simulink model "TrafficLightSystem_PhyArch_Electrical"  (R2025b)
settings: Solver=VariableStepAuto  StartTime=0.0  StopTime=10.0  RelTol=1e-3
settings Model: Creator=maric  LastModifiedBy=maric

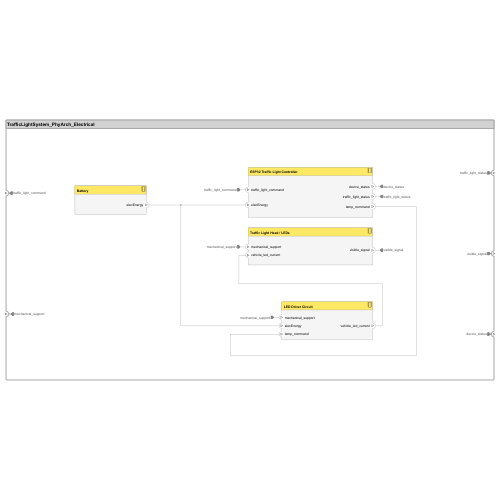
[thumbnail: Simulink's stored preview of the top-level diagram]
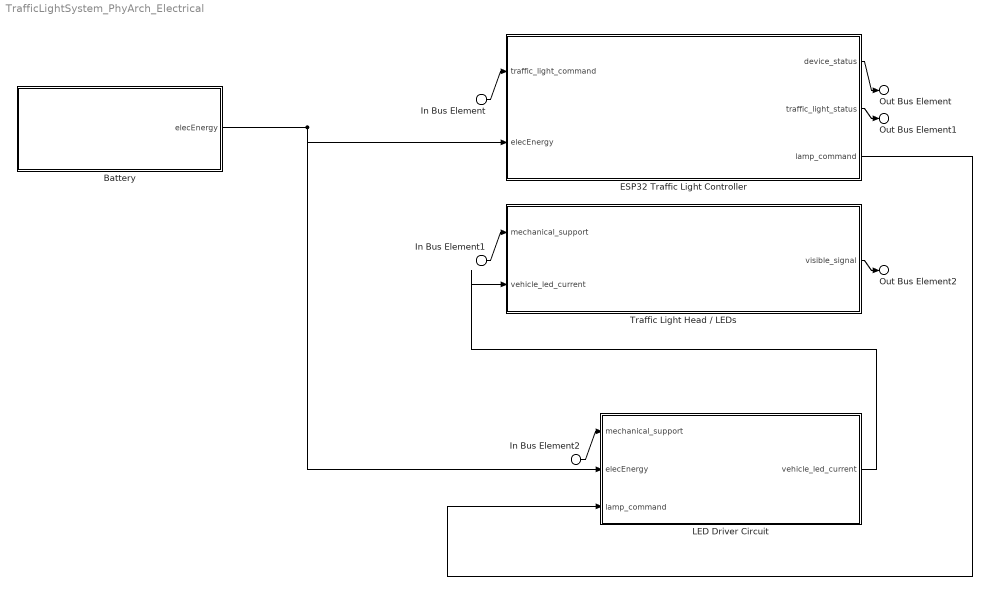
== system TrafficLightSystem_PhyArch_Electrical ==
  In Bus Element : Inport  PortName=traffic_light_command
  In Bus Element1 : Inport  Port=2  PortName=mechanical_support
  In Bus Element2 : Inport  Port=2  PortName=mechanical_support
  Battery : Subsystem
      settings: PortSchema="{\"entries\":[{\"content\":{\"headerSize\":26,\"margin\":15,\"minimumSpacing\":25,\"sides\":[{\"content\":{},\"type\":\"ConnectorPlacement.EquallySpacedRectSide\",\"uuid\":\"40d99bda-b112-4ab1-b090-826e02cba84f\"},{\"content\":{\"connectorIds\":[\"Out1\"],\"side\":\"RIGHT\"},\"type\":\"ConnectorPlacement.EquallySpacedRectSide\",\"uuid\":\"b3316996-42fc-47d8-8f6b-44af7cc05eae\"},{\"content\":{\"side\":\"TOP\"},\"type\":\"ConnectorPlacement.EquallySpacedRectSide\",\"uuid\":\"31c59802-d979-469a-9571-a9dc57a57051\"}]},\"type\":\"ConnectorPlacement.EquallySpacedConnector\",\"uuid\":\"42255f43-1755-4188-9439-b9e0458336c3\"}],\"packageUris\":[\"http://schema.mathworks.com/mf0/Connector/R2020b\"],\"version\":\"1.0\"}"
  ESP32 Traffic Light Controller : Subsystem
      settings: PortSchema="{\"entries\":[{\"content\":{\"headerSize\":26,\"margin\":15,\"minimumSpacing\":25,\"sides\":[{\"content\":{\"connectorIds\":[\"In1\",\"In2\"]},\"type\":\"ConnectorPlacement.EquallySpacedRectSide\",\"uuid\":\"fc98b1dc-f1c8-4555-a7aa-182a1386029c\"},{\"content\":{\"connectorIds\":[\"Out3\",\"Out1\",\"Out2\"],\"side\":\"RIGHT\"},\"type\":\"ConnectorPlacement.EquallySpacedRectSide\",\"uuid\":\"c81f0809-b088-4f89-b8c6-4cc559ac91af\"},{\"content\":{\"side\":\"TOP\"},\"type\":\"ConnectorPlacement.EquallySpacedRectSide\",\"uuid\":\"870463db-794f-4bc3-b33a-d9bb69248909\"}]},\"type\":\"ConnectorPlacement.EquallySpacedConnector\",\"uuid\":\"c17be9ea-9773-46b6-98e7-924568083fb3\"}],\"packageUris\":[\"http://schema.mathworks.com/mf0/Connector/R2020b\"],\"version\":\"1.0\"}"
  LED Driver Circuit : Subsystem
      settings: PortSchema="{\"entries\":[{\"content\":{\"headerSize\":26,\"margin\":15,\"minimumSpacing\":25,\"sides\":[{\"content\":{\"connectorIds\":[\"In3\",\"In2\",\"In1\"]},\"type\":\"ConnectorPlacement.EquallySpacedRectSide\",\"uuid\":\"fc98b1dc-f1c8-4555-a7aa-182a1386029c\"},{\"content\":{\"connectorIds\":[\"Out1\"],\"side\":\"RIGHT\"},\"type\":\"ConnectorPlacement.EquallySpacedRectSide\",\"uuid\":\"c81f0809-b088-4f89-b8c6-4cc559ac91af\"},{\"content\":{\"side\":\"TOP\"},\"type\":\"ConnectorPlacement.EquallySpacedRectSide\",\"uuid\":\"870463db-794f-4bc3-b33a-d9bb69248909\"}]},\"type\":\"ConnectorPlacement.EquallySpacedConnector\",\"uuid\":\"c17be9ea-9773-46b6-98e7-924568083fb3\"}],\"packageUris\":[\"http://schema.mathworks.com/mf0/Connector/R2020b\"],\"version\":\"1.0\"}"
  Traffic Light Head / LEDs : Subsystem
      settings: PortSchema="{\"entries\":[{\"content\":{\"headerSize\":26,\"margin\":15,\"minimumSpacing\":25,\"sides\":[{\"content\":{\"connectorIds\":[\"In2\",\"In1\"]},\"type\":\"ConnectorPlacement.EquallySpacedRectSide\",\"uuid\":\"fc98b1dc-f1c8-4555-a7aa-182a1386029c\"},{\"content\":{\"connectorIds\":[\"Out1\"],\"side\":\"RIGHT\"},\"type\":\"ConnectorPlacement.EquallySpacedRectSide\",\"uuid\":\"c81f0809-b088-4f89-b8c6-4cc559ac91af\"},{\"content\":{\"side\":\"TOP\"},\"type\":\"ConnectorPlacement.EquallySpacedRectSide\",\"uuid\":\"870463db-794f-4bc3-b33a-d9bb69248909\"}]},\"type\":\"ConnectorPlacement.EquallySpacedConnector\",\"uuid\":\"c17be9ea-9773-46b6-98e7-924568083fb3\"}],\"packageUris\":[\"http://schema.mathworks.com/mf0/Connector/R2020b\"],\"version\":\"1.0\"}"
  Out Bus Element1 : Outport  PortName=traffic_light_status
  Out Bus Element2 : Outport  Port=2  PortName=visible_signal
  Out Bus Element : Outport  Port=3  PortName=device_status
  wires:
  Battery/1(elecEnergy) -> ESP32 Traffic Light Controller/2(elecEnergy), LED Driver Circuit/2(elecEnergy)
  LED Driver Circuit/1(vehicle_led_current) -> Traffic Light Head / LEDs/1(vehicle_led_current)
  ESP32 Traffic Light Controller/2(lamp_command) -> LED Driver Circuit/1(lamp_command)
  In Bus Element/1 -> ESP32 Traffic Light Controller/1(traffic_light_command)
  ESP32 Traffic Light Controller/3(device_status) -> Out Bus Element/1
  ESP32 Traffic Light Controller/1(traffic_light_status) -> Out Bus Element1/1
  Traffic Light Head / LEDs/1(visible_signal) -> Out Bus Element2/1
  In Bus Element1/1 -> Traffic Light Head / LEDs/2(mechanical_support)
  In Bus Element2/1 -> LED Driver Circuit/3(mechanical_support)

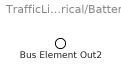
== system TrafficLightSystem_PhyArch_Electrical/Battery ==
  Bus Element Out2 : Outport  PortName=elecEnergy

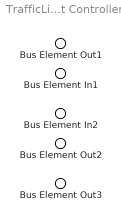
== system TrafficLightSystem_PhyArch_Electrical/ESP32 Traffic Light Controller ==
  Bus Element In1 : Inport  PortName=traffic_light_command
  Bus Element In2 : Inport  Port=2  PortName=elecEnergy
  Bus Element Out1 : Outport  PortName=traffic_light_status
  Bus Element Out2 : Outport  Port=2  PortName=lamp_command
  Bus Element Out3 : Outport  Port=3  PortName=device_status

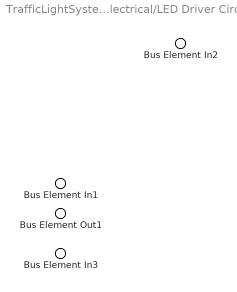
== system TrafficLightSystem_PhyArch_Electrical/LED Driver Circuit ==
  Bus Element In2 : Inport  PortName=lamp_command
  Bus Element In1 : Inport  Port=2  PortName=elecEnergy
  Bus Element In3 : Inport  Port=3  PortName=mechanical_support
  Bus Element Out1 : Outport  PortName=vehicle_led_current

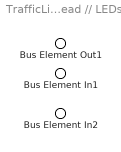
== system TrafficLightSystem_PhyArch_Electrical/Traffic Light Head // LEDs ==
  Bus Element In1 : Inport  PortName=vehicle_led_current
  Bus Element In2 : Inport  Port=2  PortName=mechanical_support
  Bus Element Out1 : Outport  PortName=visible_signal
